simulink model "OHC_IHC_Model"  (R2019a)
settings: Solver=VariableStepAuto  StartTime=0.0  StopTime=testtime  RelTol=1e-3
InitFcn:
  | OHC_IHC_Test_Parameters
StopFcn:
  | Verify_OHC_IHC_Model
values from neighbouring files (symbols this model uses):
  C1gain_norm = C1gain_norm*((CF-pimag(i))^2 + (preal(i))^2)    [OHC_IHC_Get_Parameters.m]
  C1initphase = C1initphase + atan(CF/(-rzero))-atan((CF-pimag(2*i-1))/(-preal(2*i-1)))-atan((CF+pimag(2*i-1))/(-preal(2*i-1)))    [OHC_IHC_Get_Parameters.m]
  c1LPihc = ( Cihc - 2*pi*Fcihc ) / ( Cihc + 2*pi*Fcihc )    [OHC_IHC_Get_Parameters.m]
  c1LPohc = ( Cohc - 2*pi*Fcohc ) / ( Cohc + 2*pi*Fcohc )    [OHC_IHC_Get_Parameters.m]
  C1slope = 0.1    [OHC_IHC_Get_Parameters.m]
  c2LPihc = 2*pi*Fcihc / (2*pi*Fcihc + Cihc)    [OHC_IHC_Get_Parameters.m]
  c2LPohc = 2*pi*Fcohc / (2*pi*Fcohc + Cohc)    [OHC_IHC_Get_Parameters.m]
  C2slope = 0.2    [OHC_IHC_Get_Parameters.m]
  centerfreq = 165.4*(10^((bmplace+1.2)/(35/2.1)) - 1.0)    [OHC_IHC_Get_Parameters.m]
  CF = 2*pi*cf    [OHC_IHC_Get_Parameters.m]
  cordiciterationswb = 52    [OHC_IHC_Get_Parameters.m]
  delta_phase = -2*pi*centerfreq*tdres    [OHC_IHC_Get_Parameters.m]
  fs_bilinear = 2*pi*cf/tan(2*pi*cf*tdres/2)    [OHC_IHC_Get_Parameters.m]
  gainihc = 1.0    (= 1)    [OHC_IHC_Get_Parameters.m]
  gainohc = 1.0    (= 1)    [OHC_IHC_Get_Parameters.m]
  ihcasym = 3.0    (= 3)    [OHC_IHC_Get_Parameters.m]
  m11 = 1/(C^2+5.9761e+003*C+2.5255e+007)    [OHC_IHC_Get_Parameters.m]
  m12 = -2*C^2+2*2.5255e+007    [OHC_IHC_Get_Parameters.m]
  m13 = C^2-5.9761e+003*C+2.5255e+007    [OHC_IHC_Get_Parameters.m]
  m14 = C^2+5.6665e+003*C    [OHC_IHC_Get_Parameters.m]
  m15 = -2*C^2    [OHC_IHC_Get_Parameters.m]
  m16 = C^2-5.6665e+003*C    [OHC_IHC_Get_Parameters.m]
  m21 = 1/(C^2+6.4255e+003*C+1.3975e+008)    [OHC_IHC_Get_Parameters.m]
  m22 = -2*C^2+2*1.3975e+008    [OHC_IHC_Get_Parameters.m]
  m23 = C^2-6.4255e+003*C+1.3975e+008    [OHC_IHC_Get_Parameters.m]
  m24 = C^2+5.8934e+003*C+1.7926e+008    [OHC_IHC_Get_Parameters.m]
  m25 = -2*C^2+2*1.7926e+008    [OHC_IHC_Get_Parameters.m]
  m26 = C^2-5.8934e+003*C+1.7926e+008    [OHC_IHC_Get_Parameters.m]
  m31 = 1/(C^2+2.4891e+004*C+1.2700e+009)    [OHC_IHC_Get_Parameters.m]
  m32 = -2*C^2+2*1.2700e+009    [OHC_IHC_Get_Parameters.m]
  m33 = C^2-2.4891e+004*C+1.2700e+009    [OHC_IHC_Get_Parameters.m]
  m34 = (3.1137e+003*C+6.9768e+008)    [OHC_IHC_Get_Parameters.m]
  m35 = 2*6.9768e+008    (= 1395360000)    [OHC_IHC_Get_Parameters.m]
  m36 = -3.1137e+003*C+6.9768e+008    [OHC_IHC_Get_Parameters.m]
  megainmax = 2    [OHC_IHC_Get_Parameters.m]
  minR = 0.05    [OHC_IHC_Get_Parameters.m]
  norm_gainc1 = (sqrt(C1gain_norm))/((sqrt(CF^2+rzero^2))^order_of_zero)    [OHC_IHC_Get_Parameters.m]
  ohcasym = 7.0    (= 7)    [OHC_IHC_Get_Parameters.m]
  order_of_zero = half_order_pole    (= 5)    [OHC_IHC_Get_Parameters.m]
  pimag = zeros(11,1)    [OHC_IHC_Get_Parameters.m]
  preal = zeros(11,1)    [OHC_IHC_Get_Parameters.m]
  rzero = -pzero    [OHC_IHC_Get_Parameters.m]
  s0 = 12.0    (= 12)    [OHC_IHC_Get_Parameters.m]
  s1 = 5.0    (= 5)    [OHC_IHC_Get_Parameters.m]
  shift = 1.0/(1.0+ohcasym)    (= 0.125)    [OHC_IHC_Get_Parameters.m]
  strength = (20.0e6)/(10^(corner/20))    (= 2000)    [OHC_IHC_Get_Parameters.m]
  tauwb = TauWBMax + (bmTaubm-bmTaumax)*(TauWBMax-TauWBMin)/(bmTaumax-bmTaumin)    [OHC_IHC_Get_Parameters.m]
  TauWBMax = Taumin + 0.2*(Taumax-Taumin)    [OHC_IHC_Get_Parameters.m]
  TauWBMin = TauWBMax/Taumax*Taumin    [OHC_IHC_Get_Parameters.m]
  wborder = 3    [OHC_IHC_Get_Parameters.m]
  x0 = s0*log((1.0/shift-1)/(1+exp(x1/s1)))    [OHC_IHC_Get_Parameters.m]
  x1 = 5.0    (= 5)    [OHC_IHC_Get_Parameters.m]
undefined symbols (not defined in the file or in its folder): bmTaumax, bmTaumin, cf, cihc, cohc, dfilt, Fs, jsin, norm_gainc2, tdres, wbgain
libraries: dsparch4 x5, dspsrcs4 x1
settings Model: Creator=mblun  LastModifiedBy=mblun

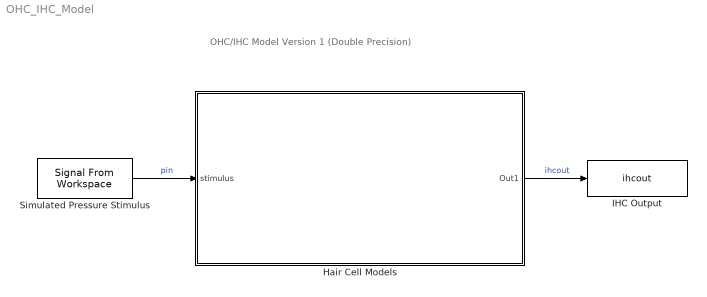
== system OHC_IHC_Model ==
  note: OHC/IHC Model Version 1 (Double Precision)
  Hair Cell Models : Subsystem
  IHC Output : ToWorkspace  VariableName=ihcout  SampleTime=-1
      settings: Save2DSignal=2-D array (concatenate along first dimension)
  Simulated Pressure Stimulus : dspsrcs4/Signal From Workspace  X=RxSignal  Ts=1/Fs  nsamps=1  OutputAfterFinalValue=Setting to zero  ignoreOrWarnInputAndFrameLengths=off  OutputFrames=off
  wires:
  Simulated Pressure Stimulus/1 -> Hair Cell Models/1(stimulus)  "pin"
  Hair Cell Models/1(Out1) -> IHC Output/1  "ihcout"

== system OHC_IHC_Model/Hair Cell Models ==
  note: IHC
  note: OHC
  stimulus : Inport
  C1 Chirp Filter : Subsystem
  C2 Wideband Filter : Subsystem
  CP Wideband Gammatone Filter : Subsystem
  Middle Ear Filter : Subsystem
  Subsystem : Subsystem
  Subsystem1 : Subsystem
  f(tauc1) : Subsystem
  Out1 : Outport
  wires:
  CP Wideband Gammatone Filter/1(output1) -> Subsystem1/1(wbout)  "wbout1"
  f(tauc1)/1(tauwb) -> CP Wideband Gammatone Filter/2(tauwb)  "tauwb"
  Subsystem1/1(tauc1) -> f(tauc1)/1(tauc1), C1 Chirp Filter/2(tauc1)  "tauc1"
  Middle Ear Filter/1(output) -> CP Wideband Gammatone Filter/3(stimulus), C1 Chirp Filter/1(meout), C2 Wideband Filter/1(stimulus)  "meout"
  stimulus/1 -> Middle Ear Filter/1(stimulus)  "pin"
  C1 Chirp Filter/1(output) -> Subsystem/2(C1filterout)  "C1filterout"
  Subsystem/1(ihcout) -> Out1/1  "ihcout"
  C2 Wideband Filter/1(output) -> Subsystem/1(C2filterout)  "C2filterout"
  f(tauc1)/2(wbgain) -> CP Wideband Gammatone Filter/1(wbgain)  "wbgain"

== system OHC_IHC_Model/Hair Cell Models/C1 Chirp Filter ==
  note: C1 Chirp Filter:
      |
      | Inputs : ME Filtered Signal (meout)
      | C1 Coefficients (a&b)
      | Normalizing Gain (norm_gain)
      |
      | Output : C1 Filtered Signal (c1filterout)
      |
      | - 10th Order IIR Bandpass Filter
      |
      | - Coefficients are determined in previous Get C1 Coefficients block
      |
      | - Implemented w/ Simulink biquad block
  note: Get C1 Coefficients
      |
      | Input : Pole-Shifting Feedback Parameter (rsigma)
      |
      | Outputs : C1 Coefficients (a&b)
      | Normalizing Gain (norm_gain)
      |
      | - Consists of various calculations to shift continuous-time pole locations according to rsigma feedback, then apply a bilinear transformation to bring the poles to the digital space before finding the coefficients for the C1 filter
  note: Calculate C1 Filter Output
      |
      | - Simply scale the output by cihc
  note: Calculate Pole-Shifting Parameter rsigma
      |
      | Input : C1 Feedback Time Constant (tauc1)
      |
      | Outputs : Pole-Shifting Parameter rsigma
      |
      | - Simple calculation to find rsigma from time constant feedback input
  meout : Inport
  tauc1 : Inport  Port=2
  C1 FIlter : Subsystem
  Calculate C1filterout : Subsystem
  Calculate rsigma : Subsystem
  Get C1 Coefficients : Subsystem
  To Workspace2 : ToWorkspace  VariableName=rsigma  SampleTime=-1
      settings: Save2DSignal=2-D array (concatenate along first dimension)
  output : Outport
  wires:
  meout/1 -> C1 FIlter/1(meout)
  C1 FIlter/1(Out1) -> Calculate C1filterout/1(C1filterouttmp)  "c1filterouttmp"
  Get C1 Coefficients/1(b0(5)) -> C1 FIlter/2(b0(5))
  Get C1 Coefficients/2(b0(3)) -> C1 FIlter/3(b0(3))
  Get C1 Coefficients/3(b0(1)) -> C1 FIlter/4(b0(1))
  Get C1 Coefficients/4(b1(5)) -> C1 FIlter/5(b1(5))
  Get C1 Coefficients/5(b1(3)) -> C1 FIlter/6(b1(3))
  Get C1 Coefficients/6(b1(1)) -> C1 FIlter/7(b1(1))
  Get C1 Coefficients/7(b2(5)) -> C1 FIlter/8(b2(5))
  Get C1 Coefficients/8(b2(3)) -> C1 FIlter/9(b2(3))
  Get C1 Coefficients/9(b2(1)) -> C1 FIlter/10(b2(1))
  Get C1 Coefficients/10(a2(5)) -> C1 FIlter/11(a2(5))
  Get C1 Coefficients/11(a2(3)) -> C1 FIlter/12(a2(3))
  Get C1 Coefficients/12(a2(1)) -> C1 FIlter/13(a2(1))
  Get C1 Coefficients/13(a1(1)) -> C1 FIlter/14(a1(1))
  Get C1 Coefficients/14(a1(3)) -> C1 FIlter/15(a1(3))
  Get C1 Coefficients/15(a1(5)) -> C1 FIlter/16(a1(5))
  Get C1 Coefficients/16(norm_gain) -> C1 FIlter/17(norm_gain)
  Calculate C1filterout/1(C1filterout) -> output/1  "C1filterout"
  Calculate rsigma/1(rsigma) -> Get C1 Coefficients/1(rsigma), To Workspace2/1  "rsigma"
  tauc1/1 -> Calculate rsigma/1(tauc1)  "tauc1"

== system OHC_IHC_Model/Hair Cell Models/C2 Wideband Filter ==
  note: C2 Wideband Filter:
      |
      | Input : ME Filtered Signal (meout)
      |
      | Output : C2 Filtered Signal (c2filterout)
      |
      | - 10th Order IIR Bandpass Filter
      |
      | - Coefficients are determined in AN_Get_Parameters init script
      |
      | - Implemented w/ Simulink biquad block
  note: Calculate C2 Filter Output:
      |
      | - Simply scale filter output
  stimulus : Inport
  Biquad Filter1 : dsparch4/Biquad Filter  FilterSource=Dialog parameters  CoeffSource=Specify via dialog  FilterObject=dfilt.df2tsos([1 0.3 0.4],[1 0.1 0.2])  IIRFiltStruct=Direct form II transposed  BiQuadCoeffs=C2coeffs  ScaleValues=1  IC=0  ICnum=0  ICden=0  a0Flag=Warning  optimizeScaleValues=on  ScaleValueMode=Specify via input port (g)  roundingMode=Floor  overflowMode=on  scaleValueFracLength=14  denProdOutputFracLength=30  denAccumFracLength=30  secondMemoryFracLength=15
      settings: SourceProductName=DSP System Toolbox
  Calculate C2filterout : Subsystem
  Gain : Gain  Gain=norm_gainc2/4
  output : Outport
  wires:
  stimulus/1 -> Biquad Filter1/1
  Biquad Filter1/1 -> Gain/1
  Gain/1 -> Calculate C2filterout/1(C2filterouttmp)  "c2filterouttmp"
  Calculate C2filterout/1(C2filterout) -> output/1  "C2filterout"

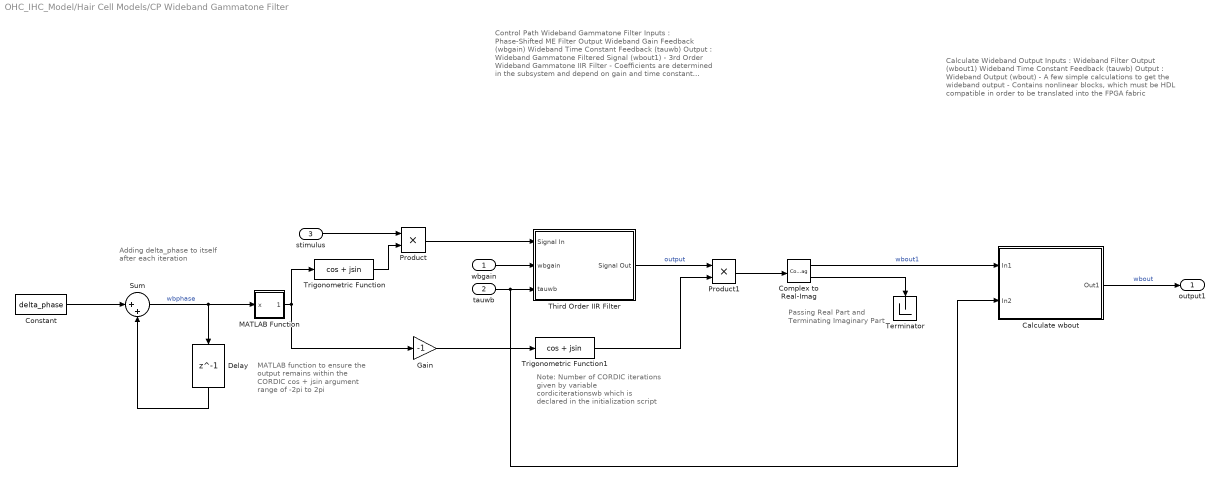
== system OHC_IHC_Model/Hair Cell Models/CP Wideband Gammatone Filter ==
  note: Passing Real Part and Terminating Imaginary Part
  note: Note: Number of CORDIC iterations given by variable cordiciterationswb which is declared in the initialization script
  note: Adding delta_phase to itself after each iteration
  note: MATLAB function to ensure the output remains within the CORDIC cos + jsin argument range of -2pi to 2pi
  note: Control Path Wideband Gammatone Filter
      |
      | Inputs : Phase-Shifted ME Filter Output
      | Wideband Gain Feedback (wbgain)
      | Wideband Time Constant Feedback (tauwb)
      |
      | Output : Wideband Gammatone Filtered Signal (wbout1)
      |
      | - 3rd Order Wideband Gammatone IIR Filter
      |
      | - Coefficients are determined in the subsystem and depend on gain and time constant feedback
      |
      | - Implemented w/ Direct Form I Block Structure
  note: Calculate Wideband Output
      |
      | Inputs : Wideband Filter Output (wbout1)
      | Wideband Time Constant Feedback (tauwb)
      |
      | Output : Wideband Output (wbout)
      |
      | - A few simple calculations to get the wideband output
      |
      | - Contains nonlinear blocks, which must be HDL compatible in order to be translated into the FPGA fabric
  wbgain : Inport
  tauwb : Inport  Port=2
  stimulus : Inport  Port=3
  Calculate wbout : Subsystem
  Complex to Real-Imag : ComplexToRealImag
  Constant : Constant  Value=delta_phase  SampleTime=-1
  Delay : Delay  DelayLength=1  InitialCondition=0  UseCircularBuffer=on
  Gain : Gain  Gain=-1
  MATLAB Function : MATLAB Function  TreatAsAtomicUnit=on
  Product : Product
  Product1 : Product
  Sum : Sum  Inputs=|++
  Terminator : Terminator
  Third Order IIR Filter : Subsystem
  Trigonometric Function : Trigonometry  Operator=cos + jsin  ApproximationMethod=CORDIC  NumberOfIterations=cordiciterationswb
  Trigonometric Function1 : Trigonometry  Operator=cos + jsin  ApproximationMethod=CORDIC  NumberOfIterations=cordiciterationswb
  output1 : Outport
  wires:
  Third Order IIR Filter/1(Signal Out) -> Product1/1  "output"
  Trigonometric Function/1 -> Product/2
  Constant/1 -> Sum/1
  stimulus/1 -> Product/1
  Product/1 -> Third Order IIR Filter/1(Signal In)
  Sum/1 -> MATLAB Function/1(x), Delay/1  "wbphase"
  Delay/1 -> Sum/2
  Product1/1 -> Complex to Real-Imag/1
  Complex to Real-Imag/1 -> Calculate wbout/1(In1)  "wbout1"
  Complex to Real-Imag/2 -> Terminator/1
  MATLAB Function/1(wbphase) -> Gain/1, Trigonometric Function/1
  Gain/1 -> Trigonometric Function1/1
  Trigonometric Function1/1 -> Product1/2
  tauwb/1 -> Calculate wbout/2(In2), Third Order IIR Filter/3(tauwb)
  wbgain/1 -> Third Order IIR Filter/2(wbgain)
  Calculate wbout/1(Out1) -> output1/1  "wbout"

== system OHC_IHC_Model/Hair Cell Models/Middle Ear Filter ==
  note: Middle Ear Filter
      |
      | Input : Pressure Stimulus Waveform (pin or px)
      |
      | Output : Filtered Signal (meout)
      |
      | - 6th Order IIR Lowpass Filter
      |
      | - Coefficients are determined in AN_Get_Parameters init script
      |
      | - Implemented w/ Simulink biquad block
  stimulus : Inport
  Biquad Filter4 : dsparch4/Biquad Filter  FilterSource=Dialog parameters  CoeffSource=Specify via dialog  FilterObject=dfilt.df2tsos([1 0.3 0.4],[1 0.1 0.2])  IIRFiltStruct=Direct form II transposed  BiQuadCoeffs=[m14*m11 m15*m11 m16*m11 1 m12*m11 m13*m11; m24*m21 m25*m21 m26*m21 1 m22*m21 m23*m21; m34*m31 m35*m31 m36*m31 1 m32*m31 m33*m31]  ScaleValues=[1 1 1 1/megainmax]  IC=0  ICnum=0  ICden=0  a0Flag=Warning  optimizeScaleValues=on  ScaleValueMode=Specify via input port (g)  roundingMode=Floor  overflowMode=on  scaleValueFracLength=14  denProdOutputFracLength=30  denAccumFracLength=30  secondMemoryFracLength=15
      settings: SourceProductName=DSP System Toolbox
  To Workspace3 : ToWorkspace  VariableName=meout  SampleTime=-1
      settings: Save2DSignal=2-D array (concatenate along first dimension)
  output : Outport
  wires:
  stimulus/1 -> Biquad Filter4/1
  Biquad Filter4/1 -> To Workspace3/1, output/1  "output"

== system OHC_IHC_Model/Hair Cell Models/Subsystem ==
  note: Sum Nonlinear Function Outputs
  note: IHC C2 Nonlinear Logarithmic Transduction Function
      |
      | Input : C2 Filtered Signal (c2filterout)
      |
      | Output : C2 Transduction Function Output (c2vihctmp)
      |
      | - Contains nonlinear blocks, which must be HDL compatible in order to be translated into the FPGA fabric
  note: IHC C1 Nonlinear Logarithmic Transduction Function
      |
      | Input : C1 Filtered Signal (c1filterout)
      |
      | Output : C1 Transduction Function Output (c1vihctmp)
      |
      | - Contains nonlinear blocks, which must be HDL compatible in order to be translated into the FPGA fabric
  note: IHC Lowpass Filter
      |
      | Input : Sum of C1 and C2 Nonlinear Outputs (ihcnonlinout)
      |
      | Output : Model Output (ihcout)
      |
      | - 7th Order IIR Lowpass Filter
      |
      | - Implemented using Simulink biquad
  C2filterout : Inport
  C1filterout : Inport  Port=2
  IHC C1 NL Logarithmic Function : Subsystem
  IHC C2 NL Logarithmic Function : Subsystem
  IHC LP Filter : Subsystem
  Sum1 : Sum  Inputs=|++
  ihcout : Outport
  wires:
  IHC C2 NL Logarithmic Function/1(output) -> Sum1/1  "c2vihctmp"
  IHC C1 NL Logarithmic Function/1(output) -> Sum1/2  "c1vihctmp"
  C1filterout/1 -> IHC C1 NL Logarithmic Function/1(stimulus)  "c1filterout"
  IHC LP Filter/1(output) -> ihcout/1  "ihcout"
  Sum1/1 -> IHC LP Filter/1(stimulus)  "ihcnonlinout"
  C2filterout/1 -> IHC C2 NL Logarithmic Function/1(stimulus)  "c2filterout"

== system OHC_IHC_Model/Hair Cell Models/Subsystem1 ==
  note: OHC Lowpass Filter
      |
      | Inputs : OHC Nonlinear Output (ohcnonlinout)
      |
      | Output : LP Filtered OHC Output (ohcout)
      |
      | - 2nd Order IIR Lowpass Filter
      |
      | - Coefficients are determined in the init script
      |
      | - Implemented w/ Simulink biquad
  note: Nonlinear Function After OHC
      |
      | Input : LP Filtered OHC Output (ohcout)
      |
      | Output : Temporary C1 Time Constant (tmptauc1)
      |
      | - Nonlinear Function designed to convert the Lowpass Filter Output to a Time Varying Constant for the C1 Filter
  note: OHC Nonlinear Boltzman Function
      |
      | Input : Wideband Output (wbout)
      |
      | Output : OHC Nonlinear Output (ohcnonlinout)
      |
      | - 2nd Order Boltzman Function
  note: Calculate C1 Time Constant
      |
      | Input : Temporary C1 Time Constant (tmptauc1)
      |
      | Output : C1 Time Constant (tauc1)
      |
      | - A simple calculation to get the final C1 time constant value
  wbout : Inport
  Calculate tauc1 : Subsystem
  NL After OHC Function : Subsystem
  OHC LP Filter : Subsystem
  OHC NL Boltzman Function : Subsystem
  To Workspace1 : ToWorkspace  VariableName=tauc1  SampleTime=-1
      settings: Save2DSignal=2-D array (concatenate along first dimension)
  tauc1 : Outport
  wires:
  wbout/1 -> OHC NL Boltzman Function/1(stimulus)  "wbout"
  NL After OHC Function/1(output) -> Calculate tauc1/1(In1)  "tmptauc1"
  OHC LP Filter/1(output) -> NL After OHC Function/1(stimulus)  "ohcout"
  OHC NL Boltzman Function/1(output) -> OHC LP Filter/1(stimulus)  "ohcnonlinout"
  Calculate tauc1/1(Out1) -> To Workspace1/1, tauc1/1  "tauc1"

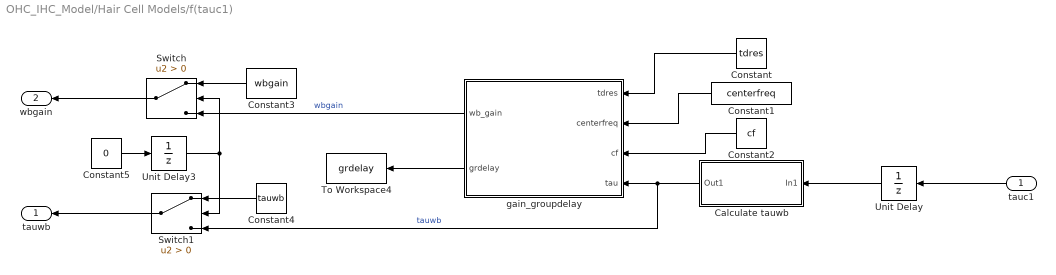
== system OHC_IHC_Model/Hair Cell Models/f(tauc1) ==
  tauc1 : Inport
  Calculate tauwb : Subsystem
  Constant : Constant  Value=tdres  SampleTime=-1
  Constant1 : Constant  Value=centerfreq  SampleTime=-1
  Constant2 : Constant  Value=cf  SampleTime=-1
  Constant3 : Constant  Value=wbgain  SampleTime=-1
  Constant4 : Constant  Value=tauwb  SampleTime=-1
  Constant5 : Constant  Value=0  SampleTime=-1
  Switch : Switch  Criteria=u2 > Threshold
  Switch1 : Switch  Criteria=u2 > Threshold
  To Workspace4 : ToWorkspace  VariableName=grdelay  SampleTime=-1
      settings: Save2DSignal=2-D array (concatenate along first dimension)
  Unit Delay : UnitDelay  SampleTime=-1  HasFrameUpgradeWarning=on
  Unit Delay3 : UnitDelay  InitialCondition=1  SampleTime=-1  HasFrameUpgradeWarning=on
  gain_groupdelay : MATLAB Function  TreatAsAtomicUnit=on
  tauwb : Outport
  wbgain : Outport  Port=2
  wires:
  Constant1/1 -> gain_groupdelay/2(centerfreq)
  tauc1/1 -> Unit Delay/1
  gain_groupdelay/1(wb_gain) -> Switch/3  "wbgain"
  Constant2/1 -> gain_groupdelay/3(cf)
  Constant/1 -> gain_groupdelay/1(tdres)
  Calculate tauwb/1(Out1) -> Switch1/3, gain_groupdelay/4(tau)  "tauwb"
  gain_groupdelay/2(grdelay) -> To Workspace4/1
  Switch/1 -> wbgain/1
  Unit Delay3/1 -> Switch/2, Switch1/2
  Switch1/1 -> tauwb/1
  Constant5/1 -> Unit Delay3/1
  Constant4/1 -> Switch1/1
  Constant3/1 -> Switch/1
  Unit Delay/1 -> Calculate tauwb/1(In1)

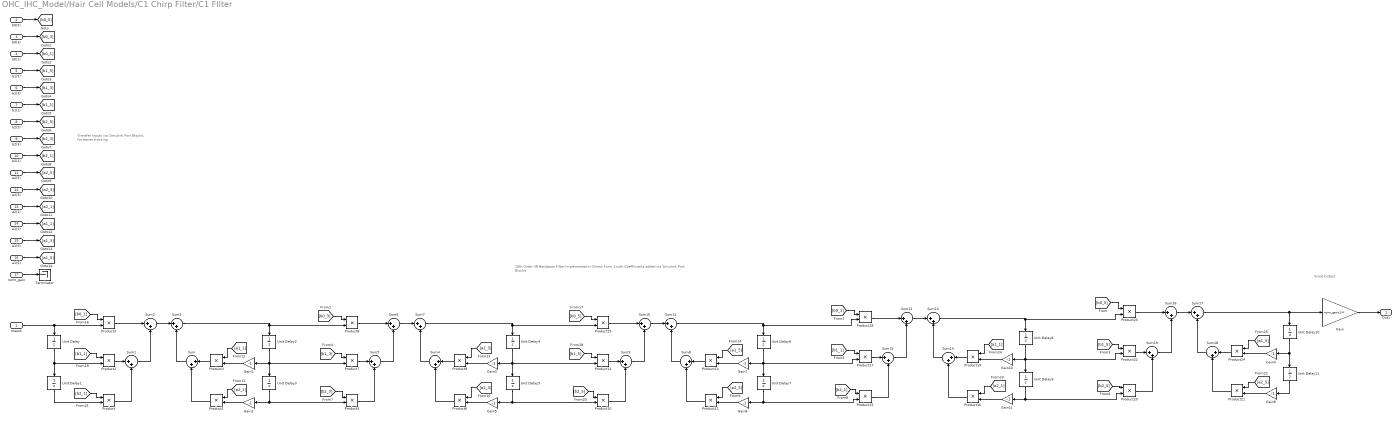
== system OHC_IHC_Model/Hair Cell Models/C1 Chirp Filter/C1 FIlter ==
  note: Transfer Inputs via Simulink Port Blocks, for easier tracking
  note: 10th Order IIR Bandpass Filter Implemented in Direct Form 1 with Coefficients added via Simulink Port Blocks
  note: Scale Output
  meout : Inport
  b0(5) : Inport  Port=2
  b0(3) : Inport  Port=3
  b0(1) : Inport  Port=4
  b1(5) : Inport  Port=5
  b1(3) : Inport  Port=6
  b1(1) : Inport  Port=7
  b2(5) : Inport  Port=8
  b2(3) : Inport  Port=9
  b2(1) : Inport  Port=10
  a2(5) : Inport  Port=11
  a2(3) : Inport  Port=12
  a2(1) : Inport  Port=13
  a1(1) : Inport  Port=14
  a1(3) : Inport  Port=15
  a1(5) : Inport  Port=16
  norm_gain : Inport  Port=17
  Gain : Gain  Gain=norm_gainc1/4
  Gain{1..5,7..11} (10 alike) : Gain  Gain=-1
  Product{,1..24} (25 alike) : Product
  Sum{,1..19} (20 alike) : Sum  Inputs=|++
  Terminator : Terminator
  Unit Delay{,1..11} (12 alike) : UnitDelay  SampleTime=-1  HasFrameUpgradeWarning=on
  Out1 : Outport
  wires:
  [a1_5] -> Product14/1
  Product15/1 -> Sum15/2
  Product16/1 -> Sum14/2
  Sum5/1 -> Sum6/2
  Sum15/1 -> Sum12/2
  Unit Delay2/1 -> Product7/2, Unit Delay3/1, Gain1/1
  Unit Delay6/1 -> Product17/2, Unit Delay7/1, Gain7/1
  [b1_3] -> Product7/1
  Sum1/1 -> Sum2/2
  [b0_1] -> Product3/1
  Product4/1 -> Sum/1
  Unit Delay8/1 -> Product22/2, Unit Delay9/1, Gain10/1
  Product12/1 -> Sum9/1
  Sum17/1 -> Unit Delay10/1, Gain/1
  Product3/1 -> Sum2/1
  [b2_3] -> Product5/1
  Sum7/1 -> Product13/2, Unit Delay4/1
  [a2_1] -> Product1/1
  [b2_1] -> Product/1
  Product24/1 -> Sum18/1
  Unit Delay3/1 -> Product5/2, Gain2/1
  Product5/1 -> Sum5/2
  Unit Delay4/1 -> Product12/2, Unit Delay5/1, Gain3/1
  Sum13/1 -> Product23/2, Unit Delay8/1
  Sum3/1 -> Product8/2, Unit Delay2/1
  Sum4/1 -> Sum7/2
  Product19/1 -> Sum14/1
  Product7/1 -> Sum5/1
  Product10/1 -> Sum9/2
  Product20/1 -> Sum19/2
  [a1_5] -> Product24/1
  Sum6/1 -> Sum7/1
  [b0_5] -> Product13/1
  [a1_3] -> Product9/1
  Product22/1 -> Sum19/1
  Product8/1 -> Sum6/1
  meout/1 -> Product3/2, Unit Delay/1
  Product2/1 -> Sum1/1
  Sum11/1 -> Product18/2, Unit Delay6/1
  Unit Delay5/1 -> Product10/2, Gain5/1
  [b1_5] -> Product12/1
  Sum2/1 -> Sum3/1
  Product11/1 -> Sum8/2
  Sum19/1 -> Sum16/2
  [b2_5] -> Product20/1
  Product14/1 -> Sum8/1
  Product18/1 -> Sum12/1
  Sum8/1 -> Sum11/2
  [b0_3] -> Product8/1
  Sum12/1 -> Sum13/1
  [b0_5] -> Product23/1
  [b0_1] -> Product18/1
  [a1_1] -> Product19/1
  [a2_5] -> Product21/1
  Unit Delay/1 -> Unit Delay1/1, Product2/2
  Product17/1 -> Sum15/1
  Unit Delay7/1 -> Product15/2, Gain8/1
  Unit Delay10/1 -> Unit Delay11/1, Gain4/1
  [a2_5] -> Product11/1
  Unit Delay11/1 -> Gain9/1
  Gain/1 -> Out1/1
  Product23/1 -> Sum16/1
  Product9/1 -> Sum4/1
  [b1_1] -> Product17/1
  Product13/1 -> Sum10/1
  Product6/1 -> Sum4/2
  Sum9/1 -> Sum10/2
  Sum16/1 -> Sum17/1
  Product21/1 -> Sum18/2
  [b1_1] -> Product2/1
  Sum18/1 -> Sum17/2
  [b1_5] -> Product22/1
  [a2_1] -> Product16/1
  [a2_3] -> Product6/1
  Sum10/1 -> Sum11/1
  [b2_5] -> Product10/1
  [b2_1] -> Product15/1
  Product/1 -> Sum1/2
  Unit Delay9/1 -> Product20/2, Gain11/1
  Sum14/1 -> Sum13/2
  [a1_1] -> Product4/1
  Sum/1 -> Sum3/2
  Unit Delay1/1 -> Product/2
  Product1/1 -> Sum/2
  b0(5)/1 -> [b0_5]
  b0(3)/1 -> [b0_3]
  b0(1)/1 -> [b0_1]
  b1(5)/1 -> [b1_5]
  b1(3)/1 -> [b1_3]
  b1(1)/1 -> [b1_1]
  b2(5)/1 -> [b2_5]
  b2(3)/1 -> [b2_3]
  b2(1)/1 -> [b2_1]
  a2(5)/1 -> [a2_5]
  a2(3)/1 -> [a2_3]
  a2(1)/1 -> [a2_1]
  a1(1)/1 -> [a1_1]
  a1(3)/1 -> [a1_3]
  a1(5)/1 -> [a1_5]
  norm_gain/1 -> Terminator/1
  Gain1/1 -> Product4/2
  Gain2/1 -> Product1/2
  Gain3/1 -> Product9/2
  Gain5/1 -> Product6/2
  Gain7/1 -> Product14/2
  Gain8/1 -> Product11/2
  Gain10/1 -> Product19/2
  Gain11/1 -> Product16/2
  Gain4/1 -> Product24/2
  Gain9/1 -> Product21/2

== system OHC_IHC_Model/Hair Cell Models/C1 Chirp Filter/Calculate C1filterout ==
  C1filterouttmp : Inport
  Gain1 : Gain  Gain=cihc
  C1filterout : Outport
  wires:
  C1filterouttmp/1 -> Gain1/1
  Gain1/1 -> C1filterout/1

== system OHC_IHC_Model/Hair Cell Models/C1 Chirp Filter/Calculate rsigma ==
  note: Note: There are multiple HDL-friendly recipricol blocks. Use this block type for highest accuracy.
  note: Calculating rsigma using time constant feedback input
  tauc1 : Inport
  Constant2 : Constant  Value=bmTaumax  SampleTime=-1
  Reciprocal : Product  Inputs=/  SaturateOnIntegerOverflow=on  RndMeth=Zero
  Reciprocal1 : Product  Inputs=/  SaturateOnIntegerOverflow=on  RndMeth=Zero
  Subtract : Sum  Inputs=+-
  rsigma : Outport
  wires:
  tauc1/1 -> Reciprocal/1
  Constant2/1 -> Reciprocal1/1
  Reciprocal/1 -> Subtract/1
  Reciprocal1/1 -> Subtract/2
  Subtract/1 -> rsigma/1

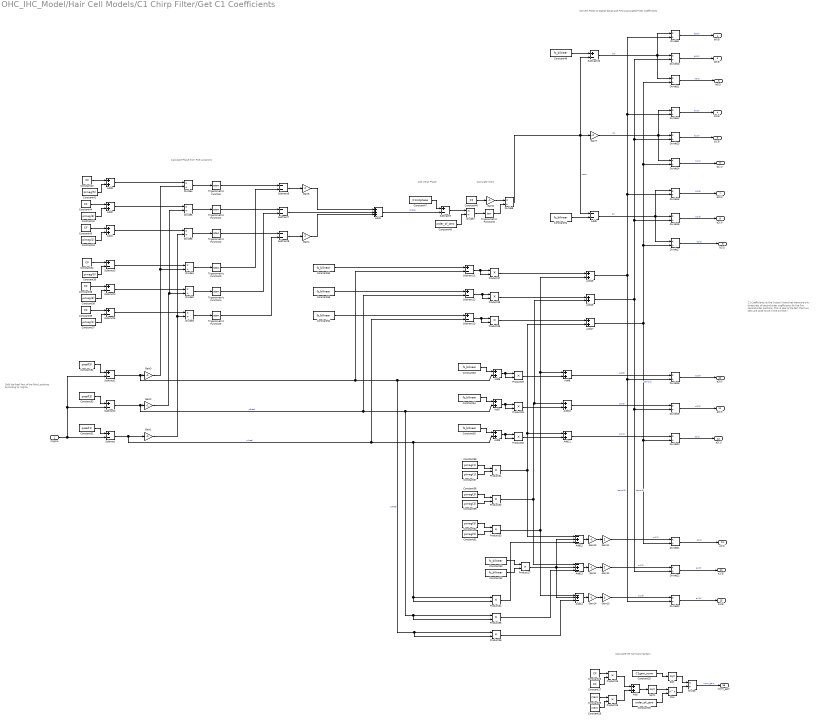
== system OHC_IHC_Model/Hair Cell Models/C1 Chirp Filter/Get C1 Coefficients ==
  note: Calculate Phase from Pole Locations
  note: Shift the Real Part of the Pole Locations according to rsigma
  note: Add Initial Phase
  note: Calculate rzero
  note: Convert Poles to Digital Spcae and Find Associated Filter Coefficients
  note: C1 Coefficients at the Output (Note that there are only three sets of second order coefficients for the five second order sections. This is due to the fact that two sets are used twice in the C1 filter)
  note: Calculate the Normalizing Gain
  rsigma : Inport
  Add{,1..3,6..11,15..17} (13 alike) : Sum
  Add12 : Sum  Inputs=-+-
  Add13 : Sum  Inputs=-+-
  Add14 : Sum  Inputs=-+-
  Add4 : Sum  Inputs=+++
  Add5 : Sum  Inputs=--
  Constant25 : Constant  Value=C1gain_norm  SampleTime=-1
  Constant{26..27,34,38..40,44..46} (9 alike) : Constant  Value=CF  SampleTime=-1
  Constant28 : Constant  Value=rzero  SampleTime=-1
  Constant29 : Constant  Value=rzero  SampleTime=-1
  Constant30 : Constant  Value=order_of_zero  SampleTime=-1
  Constant31 : Constant  Value=preal(1)  SampleTime=-1
  Constant32 : Constant  Value=preal(5)  SampleTime=-1
  Constant33 : Constant  Value=preal(3)  SampleTime=-1
  Constant{35,41,60..61} (4 alike) : Constant  Value=pimag(5)  SampleTime=-1
  Constant{36,42,58..59} (4 alike) : Constant  Value=pimag(3)  SampleTime=-1
  Constant{37,43,56..57} (4 alike) : Constant  Value=pimag(1)  SampleTime=-1
  Constant47 : Constant  Value=C1initphase  SampleTime=-1
  Constant48 : Constant  Value=order_of_zero  SampleTime=-1
  Constant{49..55,62..64} (10 alike) : Constant  Value=fs_bilinear  SampleTime=-1
  Divide{,1..23} (24 alike) : Product  Inputs=*/  SaturateOnIntegerOverflow=on  RndMeth=Zero
  Gain{1..3,6,9..10,14} (7 alike) : Gain  Gain=-1
  Gain{4..5,11..13} (5 alike) : Gain  Gain=2
  Gain7 : Gain  Gain=-2
  Pow : Math  Operator=pow  RndMeth=Zero  SaturateOnIntegerOverflow=on
  Product{25..39} (15 alike) : Product
  Sqrt : Sqrt  SaturateOnIntegerOverflow=on
  Sqrt1 : Sqrt  SaturateOnIntegerOverflow=on
  Subtract{,1..5,9..13} (11 alike) : Sum  Inputs=+-
  Subtract6 : Sum  Inputs=--
  Subtract7 : Sum  Inputs=--
  Subtract8 : Sum  Inputs=--
  Trigonometric Function{,1..5} (6 alike) : Trigonometry  Operator=atan  ApproximationMethod=CORDIC
  Trigonometric Function6 : Trigonometry  Operator=tan  ApproximationMethod=CORDIC
  b0(5) : Outport
  b0(3) : Outport  Port=2
  b0(1) : Outport  Port=3
  b1(5) : Outport  Port=4
  b1(3) : Outport  Port=5
  b1(1) : Outport  Port=6
  b2(5) : Outport  Port=7
  b2(3) : Outport  Port=8
  b2(1) : Outport  Port=9
  a2(5) : Outport  Port=10
  a2(3) : Outport  Port=11
  a2(1) : Outport  Port=12
  a1(1) : Outport  Port=13
  a1(3) : Outport  Port=14
  a1(5) : Outport  Port=15
  norm_gain : Outport  Port=16
  wires:
  Add5/1 -> Divide17/1, Divide16/1, Divide15/1  "b2"
  Constant46/1 -> Gain6/1
  Divide6/1 -> Trigonometric Function2/1
  Divide18/1 -> a2(5)/1  "a2(5)"
  Subtract9/1 -> Divide7/1
  Constant33/1 -> Subtract2/1
  Add17/1 -> Divide21/2, Divide20/2, Divide17/2, Divide11/2, Divide14/2  "temp(1)"
  Product31/1 -> Add12/1, Add17/2, Add11/1
  Gain2/1 -> Divide5/2, Divide2/2
  Subtract8/1 -> Gain4/1
  rsigma/1 -> Subtract/2, Subtract1/2, Subtract2/2
  Gain1/1 -> Divide6/2, Divide3/2
  Add12/1 -> Gain10/1
  Constant52/1 -> Product27/2
  Add13/1 -> Gain9/1
  Add15/1 -> Divide23/2, Divide18/2, Divide9/2, Divide12/2, Divide15/2  "temp(5)"
  Add14/1 -> Gain14/1
  Product27/1 -> Add14/2, Add13/2, Add12/2
  Subtract2/1 -> Subtract12/2, Product35/2, Product35/1, Add7/2, Gain2/1  "p3real"
  Subtract1/1 -> Subtract11/2, Product36/2, Product36/1, Add6/2, Gain3/1  "p5real"
  Subtract/1 -> Subtract13/2, Product34/1, Product34/2, Add8/2, Gain1/1  "p1real"
  Divide5/1 -> Trigonometric Function1/1
  Constant59/1 -> Product32/2
  Add4/1 -> Subtract9/2  "phase"
  Product30/1 -> Add11/2
  Subtract13/1 -> Product39/2, Product39/1
  Product38/1 -> Add16/1
  Product39/1 -> Add17/1
  Divide21/1 -> a1(1)/1  "a1(1)"
  Product32/1 -> Add16/2, Add10/1, Add13/1
  Subtract7/1 -> Add4/2
  Constant62/1 -> Subtract11/1
  Constant58/1 -> Product32/1
  Divide2/1 -> Trigonometric Function4/1
  Subtract10/1 -> Divide11/1, Divide10/1, Divide9/1  "b0"
  Constant31/1 -> Subtract/1
  Trigonometric Function3/1 -> Subtract6/2
  Product36/1 -> Add14/3
  Add9/1 -> Divide18/1  "a2(5)"
  Product33/1 -> Add9/1, Add15/2, Add14/1
  Constant41/1 -> Add3/2
  Constant44/1 -> Add2/1
  Gain7/1 -> Divide14/1, Divide13/1, Divide12/1  "b1"
  Product35/1 -> Add13/3
  Add16/1 -> Divide22/2, Divide19/2, Divide10/2, Divide13/2, Divide16/2  "temp(3)"
  Constant63/1 -> Subtract12/1
  Constant28/1 -> Product26/2
  Divide8/1 -> Subtract10/2, Add5/1, Gain7/1  "rzero"
  Product34/1 -> Add12/3
  Trigonometric Function4/1 -> Subtract7/2
  Trigonometric Function5/1 -> Subtract8/2
  Subtract11/1 -> Product37/2, Product37/1
  Gain11/1 -> Divide21/1  "a1(1)"
  Gain12/1 -> Divide22/1  "a1(3)"
  Constant32/1 -> Subtract1/1
  Trigonometric Function6/1 -> Divide8/2
  Divide/1 -> norm_gain/1  "norm_gain"
  Add8/1 -> Product30/2, Product30/1
  Constant40/1 -> Add3/1
  Gain6/1 -> Divide8/1
  Trigonometric Function1/1 -> Subtract7/1
  Add2/1 -> Divide5/1
  Subtract6/1 -> Gain5/1
  Gain13/1 -> Divide23/1  "a1(5)"
  Constant42/1 -> Add2/2
  Divide4/1 -> Trigonometric Function/1
  Product37/1 -> Add15/1
  Gain3/1 -> Divide4/2, Divide1/2
  Divide3/1 -> Trigonometric Function5/1
  Divide1/1 -> Trigonometric Function3/1
  Constant55/1 -> Add8/1
  Divide23/1 -> a1(5)/1  "a1(5)"
  Divide7/1 -> Trigonometric Function6/1
  Add6/1 -> Product29/2, Product29/1
  Product29/1 -> Add9/2
  Constant47/1 -> Subtract9/1
  Constant49/1 -> Subtract10/1
  Trigonometric Function2/1 -> Subtract8/1
  Subtract12/1 -> Product38/2, Product38/1
  Add3/1 -> Divide4/1
  Product25/1 -> Add/1
  Constant37/1 -> Subtract5/2
  Constant50/1 -> Product27/1
  Add11/1 -> Divide20/1  "a2(1)"
  Subtract5/1 -> Divide3/1
  Add1/1 -> Divide6/1
  Subtract4/1 -> Divide2/1
  Subtract3/1 -> Divide1/1
  Constant34/1 -> Subtract3/1
  Constant45/1 -> Add1/1
  Gain4/1 -> Add4/3
  Constant56/1 -> Product31/1
  Add7/1 -> Product28/2, Product28/1
  Constant27/1 -> Product25/2
  Gain5/1 -> Add4/1
  Constant51/1 -> Add5/2
  Product28/1 -> Add10/2
  Divide13/1 -> b1(3)/1  "b1(3)"
  Constant25/1 -> Sqrt/1
  Constant26/1 -> Product25/1
  Constant29/1 -> Product26/1
  Add/1 -> Sqrt1/1
  Sqrt/1 -> Divide/1
  Pow/1 -> Divide/2
  Sqrt1/1 -> Pow/1
  Product26/1 -> Add/2
  Constant30/1 -> Pow/2
  Constant36/1 -> Subtract4/2
  Constant39/1 -> Subtract5/1
  Constant61/1 -> Product33/2
  Constant60/1 -> Product33/1
  Constant54/1 -> Add7/1
  Constant57/1 -> Product31/2
  Constant64/1 -> Subtract13/1
  Add10/1 -> Divide19/1  "a2(3)"
  Constant38/1 -> Subtract4/1
  Trigonometric Function/1 -> Subtract6/1
  Constant35/1 -> Subtract3/2
  Constant43/1 -> Add1/2
  Constant48/1 -> Divide7/2
  Constant53/1 -> Add6/1
  Divide17/1 -> b2(1)/1  "b2(1)"
  Divide12/1 -> b1(5)/1  "b1(5)"
  Divide20/1 -> a2(1)/1  "a2(1)"
  Divide11/1 -> b0(1)/1  "b0(1)"
  Divide14/1 -> b1(1)/1  "b1(1)"
  Divide15/1 -> b2(5)/1  "b2(5)"
  Divide10/1 -> b0(3)/1  "b0(3)"
  Divide22/1 -> a1(3)/1  "a1(3)"
  Divide9/1 -> b0(5)/1  "b0(5)"
  Divide19/1 -> a2(3)/1  "a2(3)"
  Divide16/1 -> b2(3)/1  "b2(3)"
  Gain10/1 -> Gain11/1
  Gain9/1 -> Gain12/1
  Gain14/1 -> Gain13/1

== system OHC_IHC_Model/Hair Cell Models/C2 Wideband Filter/Calculate C2filterout ==
  C2filterouttmp : Inport
  Abs : Abs
  Constant : Constant  Value=cf  SampleTime=-1
  Constant1 : Constant  Value=10  SampleTime=-1
  Constant2 : Constant  Value=2e3  SampleTime=-1
  Constant3 : Constant  Value=cf  SampleTime=-1
  Divide : Product  Inputs=*/  SaturateOnIntegerOverflow=on  RndMeth=Zero
  Divide1 : Product  Inputs=*/  SaturateOnIntegerOverflow=on  RndMeth=Zero
  Product : Product
  Product1 : Product
  Product2 : Product
  C2filterout : Outport
  wires:
  C2filterouttmp/1 -> Product/1, Abs/1
  Abs/1 -> Product/2
  Product/1 -> Product1/1
  Constant/1 -> Product1/2
  Product1/1 -> Divide/1
  Constant1/1 -> Divide/2
  Product2/1 -> Divide1/1
  Constant2/1 -> Divide1/2
  Constant3/1 -> Product2/2
  Divide/1 -> Product2/1
  Divide1/1 -> C2filterout/1

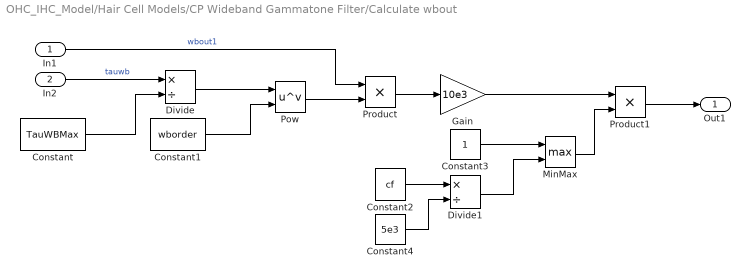
== system OHC_IHC_Model/Hair Cell Models/CP Wideband Gammatone Filter/Calculate wbout ==
  In1 : Inport
  In2 : Inport  Port=2
  Constant : Constant  Value=TauWBMax  SampleTime=-1
  Constant1 : Constant  Value=wborder  SampleTime=-1
  Constant2 : Constant  Value=cf  SampleTime=-1
  Constant3 : Constant  SampleTime=-1
  Constant4 : Constant  Value=5e3  SampleTime=-1
  Divide : Product  Inputs=*/  SaturateOnIntegerOverflow=on  RndMeth=Zero
  Divide1 : Product  Inputs=*/  SaturateOnIntegerOverflow=on  RndMeth=Zero
  Gain : Gain  Gain=10e3
  MinMax : MinMax  Function=max  Inputs=2
  Pow : Math  Operator=pow  RndMeth=Zero  SaturateOnIntegerOverflow=on
  Product : Product
  Product1 : Product
  Out1 : Outport
  wires:
  In2/1 -> Divide/1  "tauwb"
  In1/1 -> Product/1  "wbout1"
  Constant/1 -> Divide/2
  Divide/1 -> Pow/1
  Constant1/1 -> Pow/2
  Pow/1 -> Product/2
  Product/1 -> Gain/1
  Gain/1 -> Product1/1
  Divide1/1 -> MinMax/2
  Constant3/1 -> MinMax/1
  MinMax/1 -> Product1/2
  Product1/1 -> Out1/1
  Constant2/1 -> Divide1/1
  Constant4/1 -> Divide1/2

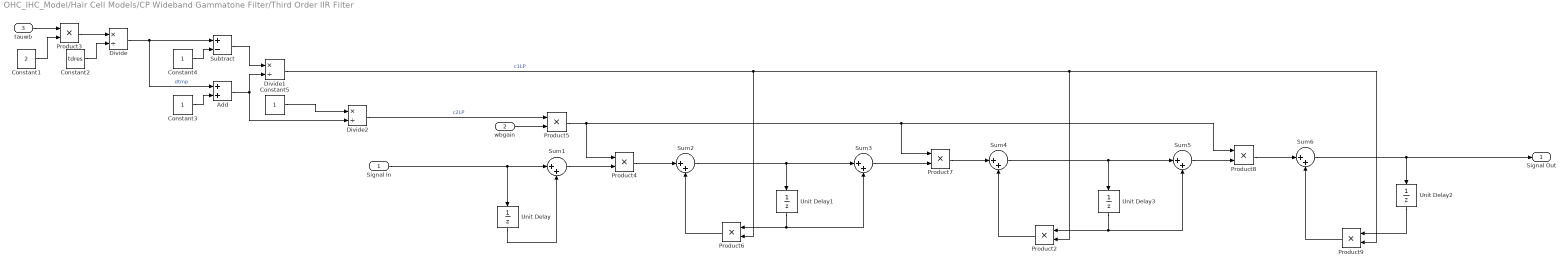
== system OHC_IHC_Model/Hair Cell Models/CP Wideband Gammatone Filter/Third Order IIR Filter ==
  Signal In : Inport
  wbgain : Inport  Port=2
  tauwb : Inport  Port=3
  Add : Sum
  Constant1 : Constant  Value=2  SampleTime=-1
  Constant2 : Constant  Value=tdres  SampleTime=-1
  Constant3 : Constant  SampleTime=-1
  Constant4 : Constant  SampleTime=-1
  Constant5 : Constant  SampleTime=-1
  Divide : Product  Inputs=*/  SaturateOnIntegerOverflow=on  RndMeth=Zero
  Divide1 : Product  Inputs=*/  SaturateOnIntegerOverflow=on  RndMeth=Zero
  Divide2 : Product  Inputs=*/  SaturateOnIntegerOverflow=on  RndMeth=Zero
  Product{2..9} (8 alike) : Product
  Subtract : Sum  Inputs=+-
  Sum{1..6} (6 alike) : Sum  Inputs=|++
  Unit Delay{,1..3} (4 alike) : UnitDelay  SampleTime=-1  HasFrameUpgradeWarning=on
  Signal Out : Outport
  wires:
  Sum6/1 -> Signal Out/1, Unit Delay2/1
  Product8/1 -> Sum6/1
  Subtract/1 -> Divide1/1
  Product2/1 -> Sum4/2
  Signal In/1 -> Unit Delay/1, Sum1/1
  Product5/1 -> Product4/1, Product7/1, Product8/1
  Constant1/1 -> Product3/2
  Divide2/1 -> Product5/1  "c2LP"
  Unit Delay/1 -> Sum1/2
  Divide/1 -> Add/1, Subtract/1  "dtmp"
  Sum3/1 -> Product7/2
  Add/1 -> Divide2/2, Divide1/2
  Sum5/1 -> Product8/2
  Unit Delay1/1 -> Sum3/2, Product6/1
  Constant5/1 -> Divide2/1
  Product7/1 -> Sum4/1
  Product9/1 -> Sum6/2
  Unit Delay3/1 -> Sum5/2, Product2/1
  Sum2/1 -> Sum3/1, Unit Delay1/1
  Product6/1 -> Sum2/2
  Sum4/1 -> Sum5/1, Unit Delay3/1
  tauwb/1 -> Product3/1
  Product3/1 -> Divide/1
  Constant4/1 -> Subtract/2
  wbgain/1 -> Product5/2
  Unit Delay2/1 -> Product9/1
  Product4/1 -> Sum2/1
  Constant2/1 -> Divide/2
  Sum1/1 -> Product4/2
  Constant3/1 -> Add/2
  Divide1/1 -> Product6/2, Product9/2, Product2/2  "c1LP"

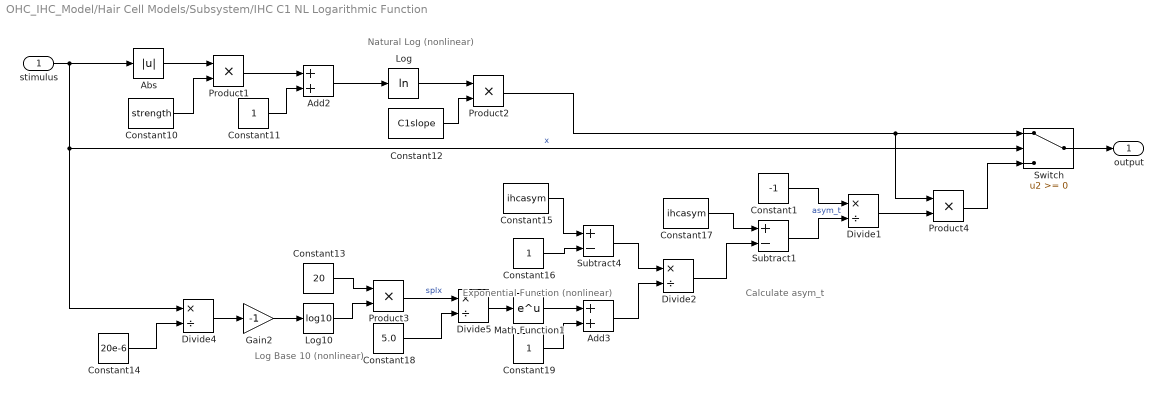
== system OHC_IHC_Model/Hair Cell Models/Subsystem/IHC C1 NL Logarithmic Function ==
  note: Calculate asym_t
  note: Log Base 10 (nonlinear)
  note: Exponential Function (nonlinear)
  note: Natural Log (nonlinear)
  stimulus : Inport
  Abs : Abs
  Add2 : Sum
  Add3 : Sum
  Constant1 : Constant  Value=-1  SampleTime=-1
  Constant10 : Constant  Value=strength  SampleTime=-1
  Constant11 : Constant  SampleTime=-1
  Constant12 : Constant  Value=C1slope  SampleTime=-1
  Constant13 : Constant  Value=20  SampleTime=-1
  Constant14 : Constant  Value=20e-6  SampleTime=-1
  Constant15 : Constant  Value=ihcasym  SampleTime=-1
  Constant16 : Constant  SampleTime=-1
  Constant17 : Constant  Value=ihcasym  SampleTime=-1
  Constant18 : Constant  Value=5.0  SampleTime=-1
  Constant19 : Constant  SampleTime=-1
  Divide{1..2,4..5} (4 alike) : Product  Inputs=*/  SaturateOnIntegerOverflow=on  RndMeth=Zero
  Gain2 : Gain  Gain=-1
  Log : Math  Operator=log  SaturateOnIntegerOverflow=on
  Log10 : Math  Operator=log10  SaturateOnIntegerOverflow=on
  Math Function1 : Math  SaturateOnIntegerOverflow=on
  Product{1..4} (4 alike) : Product
  Subtract1 : Sum  Inputs=+-
  Subtract4 : Sum  Inputs=+-
  Switch : Switch
  output : Outport
  wires:
  stimulus/1 -> Divide4/1, Switch/2, Abs/1  "x"
  Abs/1 -> Product1/1
  Constant10/1 -> Product1/2
  Constant11/1 -> Add2/2
  Product1/1 -> Add2/1
  Add2/1 -> Log/1
  Log/1 -> Product2/1
  Constant12/1 -> Product2/2
  Product2/1 -> Product4/1, Switch/1
  Constant14/1 -> Divide4/2
  Divide4/1 -> Gain2/1
  Gain2/1 -> Log10/1
  Log10/1 -> Product3/2
  Constant13/1 -> Product3/1
  Product3/1 -> Divide5/1  "splx"
  Constant15/1 -> Subtract4/1
  Constant16/1 -> Subtract4/2
  Constant18/1 -> Divide5/2
  Divide5/1 -> Math Function1/1
  Math Function1/1 -> Add3/1
  Constant19/1 -> Add3/2
  Subtract4/1 -> Divide2/1
  Add3/1 -> Divide2/2
  Constant17/1 -> Subtract1/1
  Divide2/1 -> Subtract1/2
  Subtract1/1 -> Divide1/2  "asym_t"
  Constant1/1 -> Divide1/1
  Divide1/1 -> Product4/2
  Product4/1 -> Switch/3
  Switch/1 -> output/1

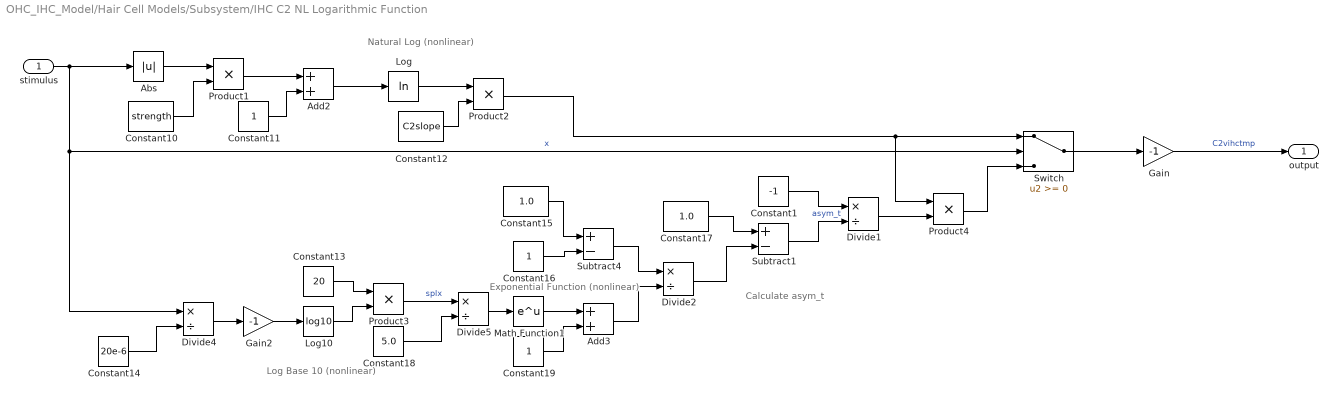
== system OHC_IHC_Model/Hair Cell Models/Subsystem/IHC C2 NL Logarithmic Function ==
  note: Calculate asym_t
  note: Exponential Function (nonlinear)
  note: Log Base 10 (nonlinear)
  note: Natural Log (nonlinear)
  stimulus : Inport
  Abs : Abs
  Add2 : Sum
  Add3 : Sum
  Constant1 : Constant  Value=-1  SampleTime=-1
  Constant10 : Constant  Value=strength  SampleTime=-1
  Constant11 : Constant  SampleTime=-1
  Constant12 : Constant  Value=C2slope  SampleTime=-1
  Constant13 : Constant  Value=20  SampleTime=-1
  Constant14 : Constant  Value=20e-6  SampleTime=-1
  Constant15 : Constant  Value=1.0  SampleTime=-1
  Constant16 : Constant  SampleTime=-1
  Constant17 : Constant  Value=1.0  SampleTime=-1
  Constant18 : Constant  Value=5.0  SampleTime=-1
  Constant19 : Constant  SampleTime=-1
  Divide{1..2,4..5} (4 alike) : Product  Inputs=*/  SaturateOnIntegerOverflow=on  RndMeth=Zero
  Gain : Gain  Gain=-1
  Gain2 : Gain  Gain=-1
  Log : Math  Operator=log  SaturateOnIntegerOverflow=on
  Log10 : Math  Operator=log10  SaturateOnIntegerOverflow=on
  Math Function1 : Math  SaturateOnIntegerOverflow=on
  Product{1..4} (4 alike) : Product
  Subtract1 : Sum  Inputs=+-
  Subtract4 : Sum  Inputs=+-
  Switch : Switch
  output : Outport
  wires:
  stimulus/1 -> Divide4/1, Switch/2, Abs/1  "x"
  Abs/1 -> Product1/1
  Constant10/1 -> Product1/2
  Constant11/1 -> Add2/2
  Product1/1 -> Add2/1
  Add2/1 -> Log/1
  Log/1 -> Product2/1
  Constant12/1 -> Product2/2
  Product2/1 -> Product4/1, Switch/1
  Constant14/1 -> Divide4/2
  Divide4/1 -> Gain2/1
  Gain2/1 -> Log10/1
  Log10/1 -> Product3/2
  Constant13/1 -> Product3/1
  Product3/1 -> Divide5/1  "splx"
  Constant15/1 -> Subtract4/1
  Constant16/1 -> Subtract4/2
  Constant18/1 -> Divide5/2
  Divide5/1 -> Math Function1/1
  Math Function1/1 -> Add3/1
  Constant19/1 -> Add3/2
  Subtract4/1 -> Divide2/1
  Add3/1 -> Divide2/2
  Constant17/1 -> Subtract1/1
  Divide2/1 -> Subtract1/2
  Subtract1/1 -> Divide1/2  "asym_t"
  Constant1/1 -> Divide1/1
  Divide1/1 -> Product4/2
  Product4/1 -> Switch/3
  Switch/1 -> Gain/1
  Gain/1 -> output/1  "C2vihctmp"

== system OHC_IHC_Model/Hair Cell Models/Subsystem/IHC LP Filter ==
  stimulus : Inport
  Biquad Filter1 : dsparch4/Biquad Filter  FilterSource=Dialog parameters  CoeffSource=Specify via dialog  FilterObject=dfilt.df2tsos([1 0.3 0.4],[1 0.1 0.2])  IIRFiltStruct=Direct form II transposed  BiQuadCoeffs=[c2LPihc c2LPihc 0 1 -c1LPihc 0; c2LPihc c2LPihc 0 1 -c1LPihc 0; c2LPihc c2LPihc 0 1 -c1LPihc 0]  ScaleValues=1  IC=0  ICnum=0  ICden=0  a0Flag=Warning  optimizeScaleValues=on  ScaleValueMode=Specify via input port (g)  roundingMode=Floor  overflowMode=on  scaleValueFracLength=14  denProdOutputFracLength=30  denAccumFracLength=30  secondMemoryFracLength=15
      settings: SourceProductName=DSP System Toolbox
  Biquad Filter4 : dsparch4/Biquad Filter  FilterSource=Dialog parameters  CoeffSource=Specify via dialog  FilterObject=dfilt.df2tsos([1 0.3 0.4],[1 0.1 0.2])  IIRFiltStruct=Direct form II transposed  BiQuadCoeffs=[gainihc*c2LPihc gainihc*c2LPihc 0 1 -c1LPihc 0; c2LPihc c2LPihc 0 1 -c1LPihc 0; c2LPihc c2LPihc 0 1 -c1LPihc 0;c2LPihc c2LPihc 0 1 -c1LPihc 0]  ScaleValues=1  IC=0  ICnum=0  ICden=0  a0Flag=Warning  optimizeScaleValues=on  ScaleValueMode=Specify via input port (g)  roundingMode=Floor  overflowMode=on  scaleValueFracLength=14  denProdOutputFracLength=30  denAccumFracLength=30  secondMemoryFracLength=15
      settings: SourceProductName=DSP System Toolbox
  output : Outport
  wires:
  stimulus/1 -> Biquad Filter4/1
  Biquad Filter4/1 -> Biquad Filter1/1  "output"
  Biquad Filter1/1 -> output/1  "output"

== system OHC_IHC_Model/Hair Cell Models/Subsystem1/Calculate tauc1 ==
  note: Calculate final Time Constant which will be fed forward into C1 filter
  In1 : Inport
  Add : Sum
  Constant : Constant  Value=cohc  SampleTime=-1
  Constant1 : Constant  Value=bmTaumin  SampleTime=-1
  Constant2 : Constant  Value=bmTaumin  SampleTime=-1
  Product : Product
  Subtract : Sum  Inputs=+-
  Out1 : Outport
  wires:
  In1/1 -> Subtract/1  "tmptauc1"
  Constant/1 -> Product/1
  Constant1/1 -> Subtract/2
  Product/1 -> Add/1
  Add/1 -> Out1/1  "tauc1"
  Subtract/1 -> Product/2
  Constant2/1 -> Add/2

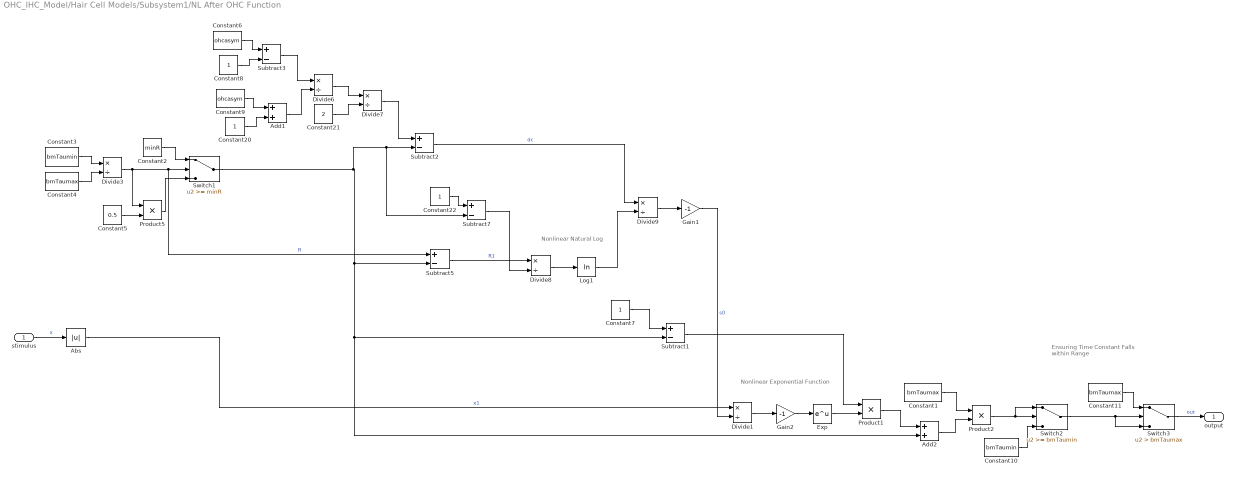
== system OHC_IHC_Model/Hair Cell Models/Subsystem1/NL After OHC Function ==
  note: Ensuring Time Constant Falls within Range
  note: Nonlinear Natural Log
  note: Nonlinear Exponential Function
  stimulus : Inport
  Abs : Abs
  Add1 : Sum
  Add2 : Sum
  Constant1 : Constant  Value=bmTaumax  SampleTime=-1
  Constant10 : Constant  Value=bmTaumin  SampleTime=-1
  Constant11 : Constant  Value=bmTaumax  SampleTime=-1
  Constant2 : Constant  Value=minR  SampleTime=-1
  Constant{7..8,20,22} (4 alike) : Constant  SampleTime=-1
  Constant21 : Constant  Value=2  SampleTime=-1
  Constant3 : Constant  Value=bmTaumin  SampleTime=-1
  Constant4 : Constant  Value=bmTaumax  SampleTime=-1
  Constant5 : Constant  Value=0.5  SampleTime=-1
  Constant6 : Constant  Value=ohcasym  SampleTime=-1
  Constant9 : Constant  Value=ohcasym  SampleTime=-1
  Divide{1,3,6..9} (6 alike) : Product  Inputs=*/  SaturateOnIntegerOverflow=on  RndMeth=Zero
  Exp : Math  SaturateOnIntegerOverflow=on
  Gain1 : Gain  Gain=-1
  Gain2 : Gain  Gain=-1
  Log1 : Math  Operator=log  SaturateOnIntegerOverflow=on
  Product1 : Product
  Product2 : Product
  Product5 : Product
  Subtract{1..3,5,7} (5 alike) : Sum  Inputs=+-
  Switch1 : Switch  Threshold=minR
  Switch2 : Switch  Threshold=bmTaumin
  Switch3 : Switch  Criteria=u2 > Threshold  Threshold=bmTaumax
  output : Outport
  wires:
  Constant3/1 -> Divide3/1
  Constant4/1 -> Divide3/2
  Divide3/1 -> Subtract5/1, Switch1/2, Product5/1  "R"
  Constant2/1 -> Switch1/1
  Constant5/1 -> Product5/2
  Product5/1 -> Switch1/3
  Switch1/1 -> Subtract7/2, Subtract2/2, Add2/2, Subtract1/2, Subtract5/2
  Constant8/1 -> Subtract3/2
  Constant6/1 -> Subtract3/1
  Constant20/1 -> Add1/2
  Constant9/1 -> Add1/1
  Subtract3/1 -> Divide6/1
  Add1/1 -> Divide6/2
  Divide6/1 -> Divide7/1
  Constant21/1 -> Divide7/2
  Divide7/1 -> Subtract2/1
  Subtract2/1 -> Divide9/1  "dc"
  Subtract5/1 -> Divide8/1  "R1"
  Constant22/1 -> Subtract7/1
  Subtract7/1 -> Divide8/2
  Divide8/1 -> Log1/1
  Log1/1 -> Divide9/2
  Divide9/1 -> Gain1/1
  Gain1/1 -> Divide1/2  "s0"
  stimulus/1 -> Abs/1  "x"
  Abs/1 -> Divide1/1  "x1"
  Constant7/1 -> Subtract1/1
  Divide1/1 -> Gain2/1
  Gain2/1 -> Exp/1
  Subtract1/1 -> Product1/1
  Exp/1 -> Product1/2
  Product1/1 -> Add2/1
  Constant1/1 -> Product2/1
  Add2/1 -> Product2/2
  Product2/1 -> Switch2/1, Switch2/2
  Constant10/1 -> Switch2/3
  Switch2/1 -> Switch3/3, Switch3/2
  Constant11/1 -> Switch3/1
  Switch3/1 -> output/1  "out"

== system OHC_IHC_Model/Hair Cell Models/Subsystem1/OHC LP Filter ==
  stimulus : Inport
  Biquad Filter4 : dsparch4/Biquad Filter  FilterSource=Dialog parameters  CoeffSource=Specify via dialog  FilterObject=dfilt.df2tsos([1 0.3 0.4],[1 0.1 0.2])  IIRFiltStruct=Direct form II transposed  BiQuadCoeffs=[gainohc*c2LPohc gainohc*c2LPohc 0 1 -c1LPohc 0; gainohc*c2LPohc gainohc*c2LPohc 0 1 -c1LPohc 0]  ScaleValues=1  IC=0  ICnum=0  ICden=0  a0Flag=Warning  optimizeScaleValues=on  ScaleValueMode=Specify via input port (g)  roundingMode=Floor  overflowMode=on  scaleValueFracLength=14  denProdOutputFracLength=30  denAccumFracLength=30  secondMemoryFracLength=15
      settings: SourceProductName=DSP System Toolbox
  output : Outport
  wires:
  stimulus/1 -> Biquad Filter4/1
  Biquad Filter4/1 -> output/1  "output"

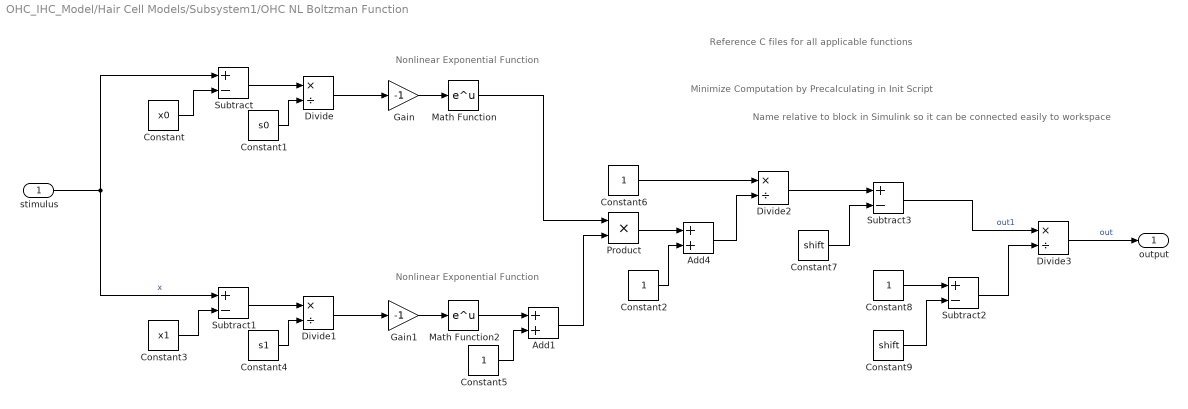
== system OHC_IHC_Model/Hair Cell Models/Subsystem1/OHC NL Boltzman Function ==
  note: Name relative to block in Simulink so it can be connected easily to workspace
  note: Minimize Computation by Precalculating in Init Script
  note: Reference C files for all applicable functions
  note: Nonlinear Exponential Function
  note: Nonlinear Exponential Function
  stimulus : Inport
  Add1 : Sum
  Add4 : Sum
  Constant : Constant  Value=x0  SampleTime=-1
  Constant1 : Constant  Value=s0  SampleTime=-1
  Constant{2,5..6,8} (4 alike) : Constant  SampleTime=-1
  Constant3 : Constant  Value=x1  SampleTime=-1
  Constant4 : Constant  Value=s1  SampleTime=-1
  Constant7 : Constant  Value=shift  SampleTime=-1
  Constant9 : Constant  Value=shift  SampleTime=-1
  Divide{,1..3} (4 alike) : Product  Inputs=*/  SaturateOnIntegerOverflow=on  RndMeth=Zero
  Gain : Gain  Gain=-1
  Gain1 : Gain  Gain=-1
  Math Function : Math  SaturateOnIntegerOverflow=on
  Math Function2 : Math  SaturateOnIntegerOverflow=on
  Product : Product
  Subtract{,1..3} (4 alike) : Sum  Inputs=+-
  output : Outport
  wires:
  Constant/1 -> Subtract/2
  stimulus/1 -> Subtract1/1, Subtract/1  "x"
  Subtract/1 -> Divide/1
  Constant1/1 -> Divide/2
  Divide/1 -> Gain/1
  Gain/1 -> Math Function/1
  Constant3/1 -> Subtract1/2
  Subtract1/1 -> Divide1/1
  Constant4/1 -> Divide1/2
  Divide1/1 -> Gain1/1
  Gain1/1 -> Math Function2/1
  Math Function2/1 -> Add1/1
  Constant5/1 -> Add1/2
  Add1/1 -> Product/2
  Constant6/1 -> Divide2/1
  Divide2/1 -> Subtract3/1
  Constant7/1 -> Subtract3/2
  Subtract3/1 -> Divide3/1  "out1"
  Constant8/1 -> Subtract2/1
  Constant9/1 -> Subtract2/2
  Subtract2/1 -> Divide3/2
  Divide3/1 -> output/1  "out"
  Math Function/1 -> Product/1
  Product/1 -> Add4/1
  Constant2/1 -> Add4/2
  Add4/1 -> Divide2/2

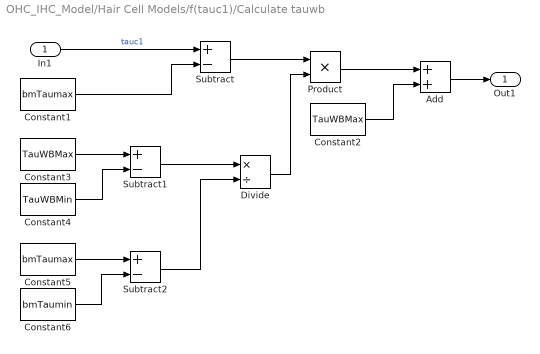
== system OHC_IHC_Model/Hair Cell Models/f(tauc1)/Calculate tauwb ==
  In1 : Inport
  Add : Sum
  Constant1 : Constant  Value=bmTaumax  SampleTime=-1
  Constant2 : Constant  Value=TauWBMax  SampleTime=-1
  Constant3 : Constant  Value=TauWBMax  SampleTime=-1
  Constant4 : Constant  Value=TauWBMin  SampleTime=-1
  Constant5 : Constant  Value=bmTaumax  SampleTime=-1
  Constant6 : Constant  Value=bmTaumin  SampleTime=-1
  Divide : Product  Inputs=*/  SaturateOnIntegerOverflow=on  RndMeth=Zero
  Product : Product
  Subtract : Sum  Inputs=+-
  Subtract1 : Sum  Inputs=+-
  Subtract2 : Sum  Inputs=+-
  Out1 : Outport
  wires:
  In1/1 -> Subtract/1  "tauc1"
  Constant1/1 -> Subtract/2
  Product/1 -> Add/1
  Subtract/1 -> Product/1
  Constant3/1 -> Subtract1/1
  Constant4/1 -> Subtract1/2
  Constant6/1 -> Subtract2/2
  Constant5/1 -> Subtract2/1
  Subtract2/1 -> Divide/2
  Subtract1/1 -> Divide/1
  Divide/1 -> Product/2
  Add/1 -> Out1/1
  Constant2/1 -> Add/2

== matlab function OHC_IHC_Model/Hair Cell Models/f(tauc1)/gain_groupdelay ==
  data: tdres input; wb_gain output; centerfreq input; cf input; tau input; grdelay output
% Matthew Blunt
% Speech % Hearing Internship
% gain_groupdelay Function
% 6/11/2019

% ---------------------------------------------------------------------- %
% NOTES: 
% ---------------------------------------------------------------------- %

% The following script is designed to replicate the gain_groupdelay
% function found in the model_IHC_BEZ2018.c file in order to verify
% functionality & implement into the Simulink model

% ---------------------------------------------------------------------- %
% CODE:
% ---------------------------------------------------------------------- %

function [wb_gain, grdelay] = gain_groupdelay(tdres, centerfreq, cf, tau)

  tmpcos = cos(2*pi*(centerfreq-cf)*tdres);
  dtmp2 = tau*2.0/tdres;
  c1LP = (dtmp2-1)/(dtmp2+1);
  c2LP = 1.0/(dtmp2+1);
  tmp1 = 1+c1LP*c1LP-2*c1LP*tmpcos;
  tmp2 = 2*c2LP*c2LP*(1+tmpcos);
  
  wb_gain = (tmp1/tmp2)^0.5;
  
  grdelay = floor((0.5-(c1LP^2-c1LP*tmpcos)/(1+c1LP^2-2*c1LP*tmpcos)));

end

== matlab function OHC_IHC_Model/Hair Cell Models/CP Wideband Gammatone Filter/MATLAB Function ==
  data: x input; wbphase output
% Matthew Blunt
% Speech % Hearing Internship
% Check Gammatone Cosine Argument
% 6/6/2019

% ---------------------------------------------------------------------- %
% NOTES: 
% ---------------------------------------------------------------------- %

% The following script is designed to work within the CP Wideband Gammatone
% Filter Simulink model in order to ensure that the argument of the
% trigonometric representation of a complex exponential remains within
% [-2pi,2pi). The function will simply take in the wb phase variable and
% output the same value in radians that falls within the range of arguments
% for the Simulink trigonometric block.

% ---------------------------------------------------------------------- %
% CODE: 
% ---------------------------------------------------------------------- %

function wbphase = WbGammaToneCosineArgCheck(x)
    while abs(x) >= 2*pi;
    if x >= 2*pi
        x = x-2*pi;
    elseif x <= -2*pi
        x = x+2*pi;
    end
    end
    wbphase = x;
end
